simulink model "non_linear_sys"  (R2021b)
settings: Solver=ode4  StartTime=0  StopTime=T_end  FixedStep=dt  RelTol=1e-3
values from neighbouring files (symbols this model uses):
  bias_Vx = 0.054595    [data.m]
  bias_Vy = 0.3    [data.m]
  delay_board_x = 0.01    [data.m]
  delay_board_y = 0.049799    [data.m]
  dt = 1e-3    (= 0.001)    [data.m]
  IC = [0.0 0.0]    [data.m]    (also in postproc2.m)
  Kbbx = (mb * g * rb^2 * rm) / ((mb * rb^2 + Jb) * Ly)    (= 0.952057453416)    [data.m]
  Kbby = (mb * g * rb^2 * rm) / ((mb * rb^2 + Jb) * Lx)    (= 1.22502497502)    [data.m]
  tau_mot_x = 0.066472    [data.m]
  tau_mot_y = 0.043174    [data.m]
  tau_sens_x = 0.025331    [data.m]
  tau_sens_y = 0.036103    [data.m]
  V2theta_x = 0.16565    [data.m]
  V2theta_y = 0.19677    [data.m]
undefined symbols (not defined in the file or in its folder): grid_pace, Kx, Kxi, Ky, Kyi, ref
libraries: simulink x4
settings Model: Creator=Daniele Oranges  LastModifiedBy=ernesto
settings DataIOCC: SaveFormat=StructureWithTime
settings OptimizationCC: BlockReduction=off  BufferReuse=off
settings DebuggingCC: AlgebraicLoopMsg=none  UnconnectedInputMsg=none  UnconnectedOutputMsg=none  UnconnectedLineMsg=none
settings ExplorerConfigSet: SimMechanicsOpenEditorOnUpdate=off

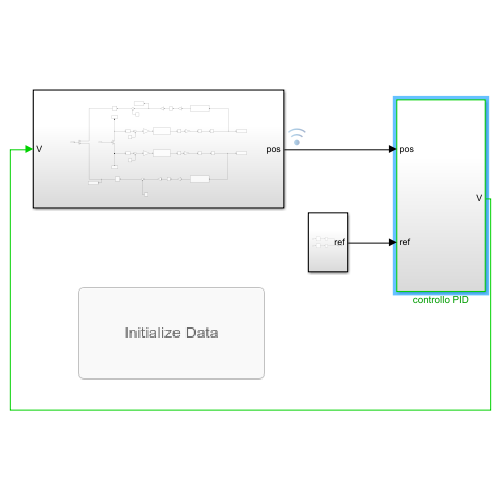
[thumbnail: Simulink's stored preview of the top-level diagram]
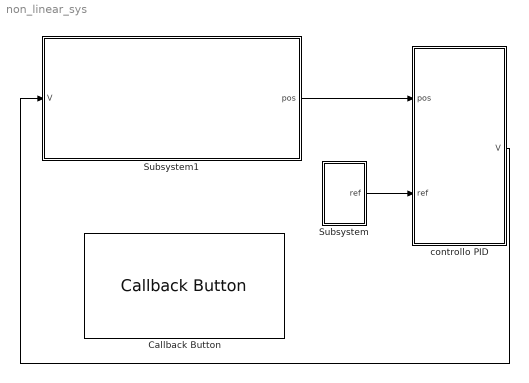
== system non_linear_sys ==
  Callback Button : CallbackButton  ButtonText=Initialize Data
      settings: ClickFcn=|
      | clear
      | data
  Subsystem : Subsystem
  Subsystem1 : Subsystem
  controllo PID : Subsystem  SystemSampleTime=0.01
  wires:
  Subsystem/1(ref) -> controllo PID/2("ref ")
  Subsystem1/1(pos) -> controllo PID/1("pos ")
  controllo PID/1(V) -> Subsystem1/1(V)

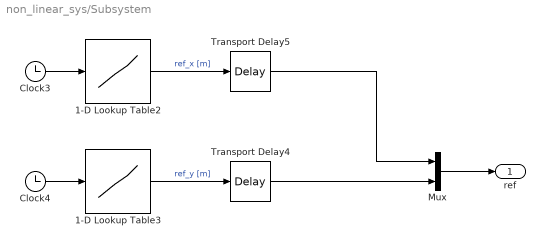
== system non_linear_sys/Subsystem ==
  1-D Lookup Table2 : Lookup_n-D  NumberOfTableDimensions=1  BreakpointsForDimension1=ref.x.t  Table=ref.x.v  InternalRulePriority=Speed  RndMeth=Simplest  InputSameDT=on
  1-D Lookup Table3 : Lookup_n-D  NumberOfTableDimensions=1  BreakpointsForDimension1=ref.y.t  Table=ref.y.v  InternalRulePriority=Speed  RndMeth=Simplest  InputSameDT=on
  Clock3 : Clock
  Clock4 : Clock
  Mux : Mux  Inputs=2
  Transport Delay4 : TransportDelay  DelayTime=dt
  Transport Delay5 : TransportDelay  DelayTime=dt
  ref : Outport
  wires:
  Transport Delay5/1 -> Mux/1
  1-D Lookup Table2/1 -> Transport Delay5/1  "ref_x [m]"
  1-D Lookup Table3/1 -> Transport Delay4/1  "ref_y [m]"
  Clock4/1 -> 1-D Lookup Table3/1
  Clock3/1 -> 1-D Lookup Table2/1
  Transport Delay4/1 -> Mux/2
  Mux/1 -> ref/1

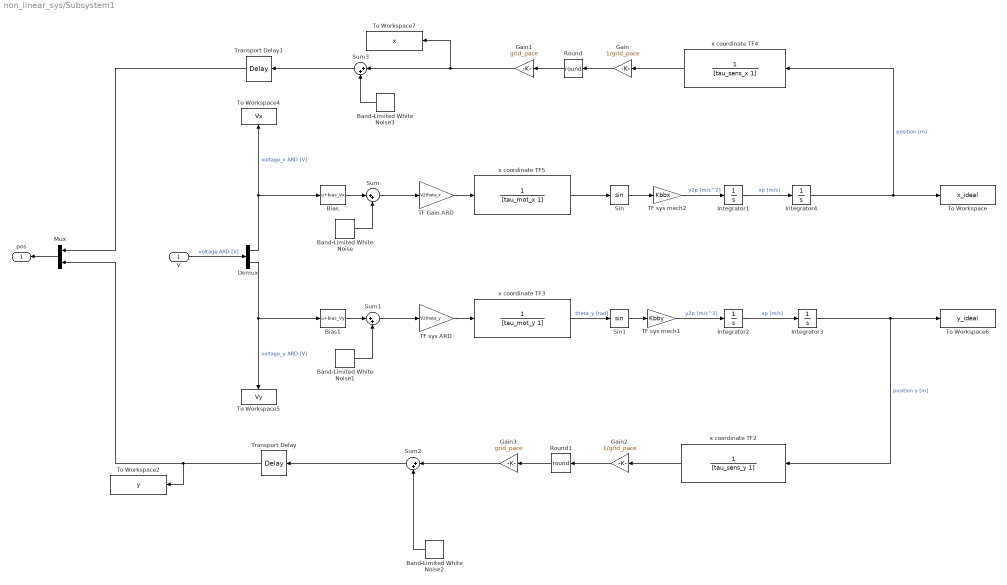
== system non_linear_sys/Subsystem1 ==
  V : Inport
  Band-Limited White Noise : simulink/Sources/Band-Limited White Noise  Cov=Ntension  Ts=dt  seed=[23341]
  Band-Limited White Noise1 : simulink/Sources/Band-Limited White Noise  Cov=Ntension  Ts=dt  seed=[23341]
  Band-Limited White Noise2 : simulink/Sources/Band-Limited White Noise  Cov=Nsensor  Ts=0.05  seed=[23341]
  Band-Limited White Noise3 : simulink/Sources/Band-Limited White Noise  Cov=Nsensor  Ts=0.05  seed=[23341]
  Bias : Bias  Bias=bias_Vx
  Bias1 : Bias  Bias=bias_Vy
  Demux : Demux  Outputs=2
  Gain : Gain  Gain=1/grid_pace
  Gain1 : Gain  Gain=grid_pace
  Gain2 : Gain  Gain=1/grid_pace
  Gain3 : Gain  Gain=grid_pace
  Integrator1 : Integrator
  Integrator2 : Integrator
  Integrator3 : Integrator  InitialCondition=IC(2)
  Integrator4 : Integrator  InitialCondition=IC(1)
  Mux : Mux  Inputs=2
  Round : Rounding  Operator=round
  Round1 : Rounding  Operator=round
  Sin : Trigonometry
  Sin1 : Trigonometry
  Sum{,1..3} (4 alike) : Sum  Inputs=|++
  TF Gain ARD : Gain  Gain=V2theta_x
  TF sys ARD : Gain  Gain=V2theta_y
  TF sys mech1 : Gain  Gain=Kbby
  TF sys mech2 : Gain  Gain=Kbbx
  To Workspace : ToWorkspace  VariableName=x_ideal  SaveFormat=Timeseries  SampleTime=-1
  To Workspace2 : ToWorkspace  VariableName=y  SaveFormat=Timeseries  SampleTime=-1
  To Workspace4 : ToWorkspace  VariableName=Vx  SaveFormat=Timeseries  SampleTime=-1
  To Workspace5 : ToWorkspace  VariableName=Vy  SaveFormat=Timeseries  SampleTime=-1
  To Workspace6 : ToWorkspace  VariableName=y_ideal  SaveFormat=Timeseries  SampleTime=-1
  To Workspace7 : ToWorkspace  VariableName=x  SaveFormat=Timeseries  SampleTime=-1
  Transport Delay : TransportDelay  DelayTime=delay_board_y
  Transport Delay1 : TransportDelay  DelayTime=delay_board_x
  x coordinate TF2 : TransferFcn  Denominator=[tau_sens_y 1]
  x coordinate TF3 : TransferFcn  Denominator=[tau_mot_y 1]
  x coordinate TF4 : TransferFcn  Denominator=[tau_sens_x 1]
  x coordinate TF5 : TransferFcn  Denominator=[tau_mot_x 1]
  pos : Outport
  wires:
  Demux/1 -> To Workspace4/1, Bias/1  "voltage_x ARD [V]"
  Integrator4/1 -> To Workspace/1, x coordinate TF4/1  "position [m]"
  Demux/2 -> To Workspace5/1, Bias1/1  "voltage_y ARD [V]"
  Integrator3/1 -> To Workspace6/1, x coordinate TF2/1  "position y [m]"
  V/1 -> Demux/1  "voltage ARD [V]"
  Mux/1 -> pos/1
  x coordinate TF5/1 -> Sin/1
  TF Gain ARD/1 -> x coordinate TF5/1
  x coordinate TF3/1 -> Sin1/1  "theta_y [rad]"
  TF sys ARD/1 -> x coordinate TF3/1
  Integrator2/1 -> Integrator3/1  "xp [m/s]"
  TF sys mech1/1 -> Integrator2/1  "y2p [m/s^2]"
  Integrator1/1 -> Integrator4/1  "xp [m/s]"
  TF sys mech2/1 -> Integrator1/1  "y2p [m/s^2]"
  Gain/1 -> Round/1
  Round/1 -> Gain1/1
  x coordinate TF4/1 -> Gain/1
  Gain1/1 -> Sum3/1, To Workspace7/1
  Bias/1 -> Sum/1
  Sum/1 -> TF Gain ARD/1
  Band-Limited White Noise/1 -> Sum/2
  Round1/1 -> Gain3/1
  Gain2/1 -> Round1/1
  x coordinate TF2/1 -> Gain2/1
  Band-Limited White Noise1/1 -> Sum1/2
  Bias1/1 -> Sum1/1
  Sum1/1 -> TF sys ARD/1
  Sin/1 -> TF sys mech2/1
  Sin1/1 -> TF sys mech1/1
  Transport Delay1/1 -> Mux/1
  Transport Delay/1 -> Mux/2, To Workspace2/1
  Band-Limited White Noise2/1 -> Sum2/2
  Gain3/1 -> Sum2/1
  Sum2/1 -> Transport Delay/1
  Band-Limited White Noise3/1 -> Sum3/2
  Sum3/1 -> Transport Delay1/1

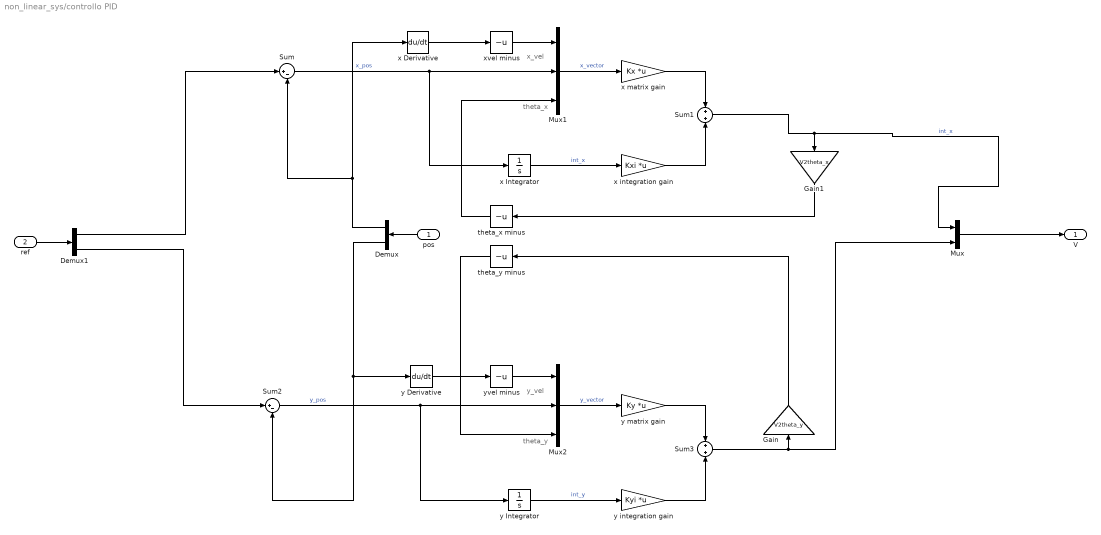
== system non_linear_sys/controllo PID ==
  note: theta_x
  note: x_vel
  note: theta_y
  note: y_vel
  "pos " : Inport
  "ref " : Inport  Port=2
  Demux : Demux  Outputs=2
  Demux1 : Demux  Outputs=2
  Gain : Gain  Gain=V2theta_y
  Gain1 : Gain  Gain=V2theta_x
  Mux : Mux  Inputs=2
  Mux1 : Mux  Inputs=3
  Mux2 : Mux  Inputs=3
  Sum : Sum  Inputs=|+-
  Sum1 : Sum  Inputs=+|+
  Sum2 : Sum  Inputs=|+-
  Sum3 : Sum  Inputs=+|+
  theta_x minus : UnaryMinus
  theta_y minus : UnaryMinus
  x Derivative : Derivative
  x Integrator : Integrator
  x integration gain : Gain  Gain=Kxi  Multiplication=Matrix(K*u)
  x matrix gain : Gain  Gain=Kx  Multiplication=Matrix(K*u)
  xvel minus : UnaryMinus
  y Derivative : Derivative
  y Integrator : Integrator
  y integration gain : Gain  Gain=Kyi  Multiplication=Matrix(K*u)
  y matrix gain : Gain  Gain=Ky  Multiplication=Matrix(K*u)
  yvel minus : UnaryMinus
  V : Outport
  wires:
  "ref "/1 -> Demux1/1
  "pos "/1 -> Demux/1
  Mux/1 -> V/1
  Demux1/1 -> Sum/1
  Demux/1 -> x Derivative/1, Sum/2
  x Derivative/1 -> xvel minus/1
  Sum/1 -> x Integrator/1, Mux1/2  "x_pos"
  Mux1/1 -> x matrix gain/1  "x_vector"
  x Integrator/1 -> x integration gain/1  "int_x"
  x matrix gain/1 -> Sum1/1
  x integration gain/1 -> Sum1/2
  y Derivative/1 -> yvel minus/1
  Sum2/1 -> y Integrator/1, Mux2/2  "y_pos"
  Mux2/1 -> y matrix gain/1  "y_vector"
  y Integrator/1 -> y integration gain/1  "int_y"
  y matrix gain/1 -> Sum3/1
  y integration gain/1 -> Sum3/2
  Demux1/2 -> Sum2/1
  Demux/2 -> y Derivative/1, Sum2/2
  Sum3/1 -> Gain/1, Mux/2
  theta_x minus/1 -> Mux1/3
  theta_y minus/1 -> Mux2/3
  xvel minus/1 -> Mux1/1
  yvel minus/1 -> Mux2/1
  Gain/1 -> theta_y minus/1
  Gain1/1 -> theta_x minus/1
  Sum1/1 -> Mux/1, Gain1/1  "int_x"
